simulink model "CSD_Segway_Nonlinear"  (R2018b)
settings: Solver=ode5  StartTime=0.0  StopTime=10  FixedStep=1e-4  RelTol=1e-3
values from neighbouring files (symbols this model uses):
  alpha = n * k_t / R_m    (= 0.0446559297218)    [CSD_project.m]
  beta = n * k_t * k_b /R_m + f_m    (= 0.0270286969253)    [CSD_project.m]
  f_w = 0    [CSD_project.m]
  g = 9.81    [CSD_project.m]
  J_m = 10^(-5)    (= 1e-05)    [CSD_project.m]
  K = place(A, B, 1e2*[-5,      -1, -0.8, -0.8,      -2e-2, -2e-2])    [CSD_project.m]
  L = 0.125    [CSD_project.m]
  M = 0.6    [CSD_project.m]
  m_1 = (2 * m + M) * R^2 + 2 * J_w + 2 * n^2 * J_m    (= 0.00056096)    [CSD_project.m]
  m_3 = M * L^2 + J_psi + 2 * n^2 * J_m    (= 0.01252)    [CSD_project.m]
  m_4 = m * W^2 /2 + J_phi + W^2 / 2 / R^2 * (J_w + n^2 * J_m)    (= 0.00149726)    [CSD_project.m]
  n = 1    [CSD_project.m]
  R = 0.028    [CSD_project.m]
  W = 0.126    [CSD_project.m]
settings Model: Creator=sh  LastModifiedBy=sh

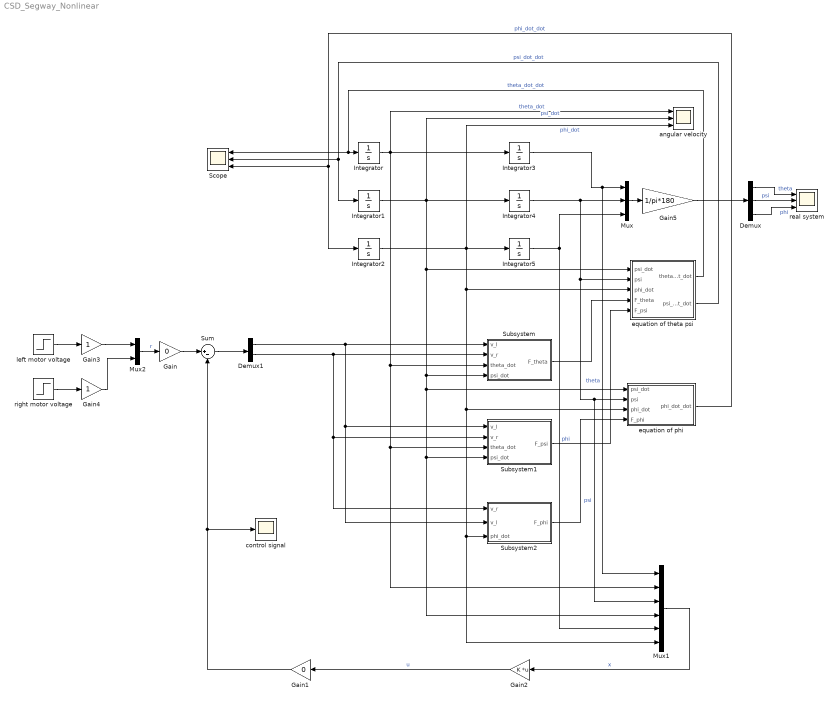
== system CSD_Segway_Nonlinear ==
  Demux : Demux  Outputs=3
  Demux1 : Demux  Outputs=2
  Gain : Gain  Gain=0
  Gain1 : Gain  Gain=0
  Gain2 : Gain  Gain=K  Multiplication=Matrix(K*u)
  Gain3 : Gain
  Gain4 : Gain
  Gain5 : Gain  Gain=1/pi*180
  Integrator : Integrator
  Integrator1 : Integrator
  Integrator2 : Integrator
  Integrator3 : Integrator  InitialCondition=pi
  Integrator4 : Integrator  InitialCondition=pi/36
  Integrator5 : Integrator  InitialCondition=pi/2
  Mux : Mux  Inputs=3
  Mux1 : Mux  Inputs=6
  Mux2 : Mux  Inputs=2
  Scope : Scope  NumInputPorts=3
  Subsystem : Subsystem
  Subsystem1 : Subsystem
  Subsystem2 : Subsystem
  Sum : Sum  Inputs=|+-
  angular velocity : Scope  NumInputPorts=3
  control signal : Scope
  equation of phi : Subsystem
  equation of theta psi : Subsystem
  left motor voltage : Step  SampleTime=0
  real system : Scope  NumInputPorts=3
  right motor voltage : Step  SampleTime=0
  wires:
  Integrator3/1 -> Mux1/1, Mux/1  "theta"
  Subsystem2/1(F_phi) -> equation of phi/4(F_phi)
  Subsystem/1(F_theta) -> equation of theta psi/4(F_theta)
  Integrator2/1 -> angular velocity/3, equation of theta psi/3(phi_dot), equation of phi/3(phi_dot), Mux1/6, Subsystem2/3(phi_dot), Integrator5/1  "phi_dot"
  Integrator/1 -> angular velocity/1, Mux1/2, Subsystem1/3(theta_dot), Subsystem/3(theta_dot), Integrator3/1  "theta_dot"
  equation of theta psi/2(psi_dot_dot) -> Integrator1/1, Scope/2  "psi_dot_dot"
  equation of theta psi/1(theta_dot_dot) -> Scope/1, Integrator/1  "theta_dot_dot"
  Integrator1/1 -> angular velocity/2, equation of theta psi/1(psi_dot), equation of phi/1(psi_dot), Mux1/4, Subsystem1/4(psi_dot), Subsystem/4(psi_dot), Integrator4/1  "psi_dot"
  Demux1/2 -> Subsystem2/1(v_r), Subsystem1/2(v_r), Subsystem/2(v_r)
  equation of phi/1(phi_dot_dot) -> Integrator2/1, Scope/3  "phi_dot_dot"
  Integrator4/1 -> Mux/2, Mux1/3, equation of phi/2(psi), equation of theta psi/2(psi)  "psi"
  Demux1/1 -> Subsystem1/1(v_l), Subsystem2/2(v_l), Subsystem/1(v_l)
  Subsystem1/1(F_psi) -> equation of theta psi/5(F_psi)
  Integrator5/1 -> Mux/3, Mux1/5  "phi"
  Mux1/1 -> Gain2/1  "x"
  Mux2/1 -> Gain/1  "r"
  left motor voltage/1 -> Gain3/1
  right motor voltage/1 -> Gain4/1
  Sum/1 -> Demux1/1
  Gain2/1 -> Gain1/1  "u"
  Gain/1 -> Sum/1
  Gain1/1 -> control signal/1, Sum/2
  Gain3/1 -> Mux2/1
  Gain4/1 -> Mux2/2
  Demux/1 -> real system/1  "theta"
  Demux/2 -> real system/2  "psi"
  Demux/3 -> real system/3  "phi"
  Mux/1 -> Gain5/1
  Gain5/1 -> Demux/1

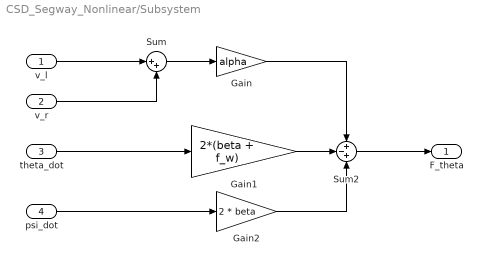
== system CSD_Segway_Nonlinear/Subsystem ==
  v_l : Inport
  v_r : Inport  Port=2
  theta_dot : Inport  Port=3
  psi_dot : Inport  Port=4
  Gain : Gain  Gain=alpha
  Gain1 : Gain  Gain=2*(beta + f_w)
  Gain2 : Gain  Gain=2 * beta
  Sum : Sum  Inputs=|++
  Sum2 : Sum  Inputs=+-+
  F_theta : Outport
  wires:
  v_l/1 -> Sum/1
  theta_dot/1 -> Gain1/1
  v_r/1 -> Sum/2
  Sum2/1 -> F_theta/1
  Gain1/1 -> Sum2/2
  Gain/1 -> Sum2/1
  Sum/1 -> Gain/1
  psi_dot/1 -> Gain2/1
  Gain2/1 -> Sum2/3

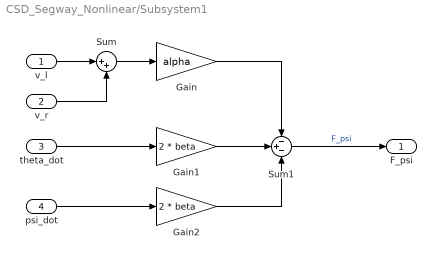
== system CSD_Segway_Nonlinear/Subsystem1 ==
  v_l : Inport
  v_r : Inport  Port=2
  theta_dot : Inport  Port=3
  psi_dot : Inport  Port=4
  Gain : Gain  Gain=alpha
  Gain1 : Gain  Gain=2 * beta
  Gain2 : Gain  Gain=2 * beta
  Sum : Sum  Inputs=|++
  Sum1 : Sum  Inputs=-+-
  F_psi : Outport
  wires:
  psi_dot/1 -> Gain2/1
  v_l/1 -> Sum/1
  Sum/1 -> Gain/1
  Sum1/1 -> F_psi/1  "F_psi"
  theta_dot/1 -> Gain1/1
  Gain/1 -> Sum1/1
  v_r/1 -> Sum/2
  Gain2/1 -> Sum1/3
  Gain1/1 -> Sum1/2

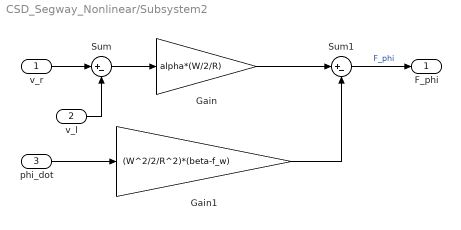
== system CSD_Segway_Nonlinear/Subsystem2 ==
  v_r : Inport
  v_l : Inport  Port=2
  phi_dot : Inport  Port=3
  Gain : Gain  Gain=alpha*(W/2/R)
  Gain1 : Gain  Gain=(W^2/2/R^2)*(beta-f_w)
  Sum : Sum  Inputs=|+-
  Sum1 : Sum  Inputs=|+-
  F_phi : Outport
  wires:
  Sum1/1 -> F_phi/1  "F_phi"
  phi_dot/1 -> Gain1/1
  v_l/1 -> Sum/2
  v_r/1 -> Sum/1
  Sum/1 -> Gain/1
  Gain/1 -> Sum1/1
  Gain1/1 -> Sum1/2

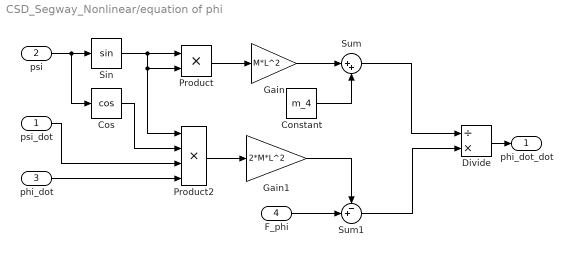
== system CSD_Segway_Nonlinear/equation of phi ==
  psi_dot : Inport
  psi : Inport  Port=2
  phi_dot : Inport  Port=3
  F_phi : Inport  Port=4
  Constant : Constant  Value=m_4
  Cos : Trigonometry  Operator=cos
  Divide : Product  Inputs=/*
  Gain : Gain  Gain=M*L^2
  Gain1 : Gain  Gain=2*M*L^2
  Product : Product
  Product2 : Product  Inputs=4
  Sin : Trigonometry
  Sum : Sum  Inputs=|++
  Sum1 : Sum  Inputs=-+|
  phi_dot_dot : Outport
  wires:
  psi_dot/1 -> Product2/3
  F_phi/1 -> Sum1/2
  Gain/1 -> Sum/1
  Constant/1 -> Sum/2
  Product2/1 -> Gain1/1
  Sum/1 -> Divide/1
  Gain1/1 -> Sum1/1
  psi/1 -> Cos/1, Sin/1
  Product/1 -> Gain/1
  Sum1/1 -> Divide/2
  phi_dot/1 -> Product2/4
  Cos/1 -> Product2/2
  Divide/1 -> phi_dot_dot/1
  Sin/1 -> Product/2, Product2/1, Product/1

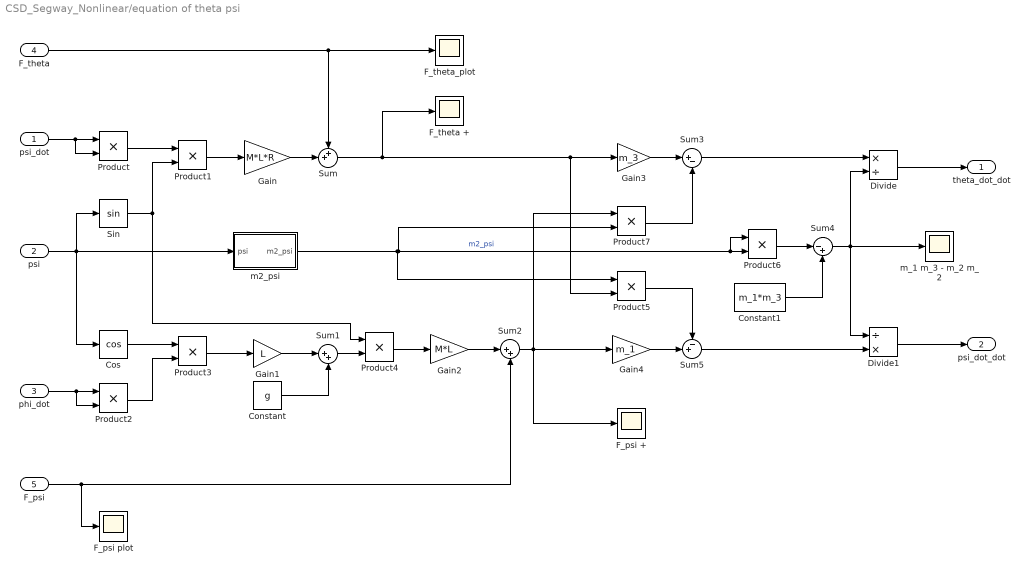
== system CSD_Segway_Nonlinear/equation of theta psi ==
  psi_dot : Inport
  psi : Inport  Port=2
  phi_dot : Inport  Port=3
  F_theta : Inport  Port=4
  F_psi : Inport  Port=5
  Constant : Constant  Value=g
  Constant1 : Constant  Value=m_1*m_3
  Cos : Trigonometry  Operator=cos
  Divide : Product  Inputs=*/
  Divide1 : Product  Inputs=/*
  "F_psi + " : Scope
  F_psi plot : Scope
  F_theta + : Scope
  F_theta_plot : Scope
  Gain : Gain  Gain=M*L*R
  Gain1 : Gain  Gain=L
  Gain2 : Gain  Gain=M*L
  Gain3 : Gain  Gain=m_3
  Gain4 : Gain  Gain=m_1
  Product{,1..7} (8 alike) : Product
  Sin : Trigonometry
  Sum : Sum  Inputs=++|
  Sum1 : Sum  Inputs=|++
  Sum2 : Sum  Inputs=|++
  Sum3 : Sum  Inputs=|+-
  Sum4 : Sum  Inputs=|-+
  Sum5 : Sum  Inputs=-+|
  m2_psi : Subsystem
  m_1 m_3 - m_2 m_2 : Scope
  theta_dot_dot : Outport
  psi_dot_dot : Outport  Port=2
  wires:
  Product2/1 -> Product3/2
  Product4/1 -> Gain2/1
  Gain2/1 -> Sum2/1
  Gain1/1 -> Sum1/1
  psi/1 -> Cos/1, m2_psi/1(psi), Sin/1
  F_psi/1 -> F_psi plot/1, Sum2/2
  Product3/1 -> Gain1/1
  Sum1/1 -> Product4/2
  phi_dot/1 -> Product2/2, Product2/1
  Product1/1 -> Gain/1
  psi_dot/1 -> Product/2, Product/1
  Cos/1 -> Product3/1
  Product/1 -> Product1/1
  Constant/1 -> Sum1/2
  Sum/1 -> F_theta +/1, Product5/2, Gain3/1
  Sum2/1 -> "F_psi + "/1, Product7/1, Gain4/1
  Gain3/1 -> Sum3/1
  Product7/1 -> Sum3/2
  Sum3/1 -> Divide/1
  Product6/1 -> Sum4/1
  Constant1/1 -> Sum4/2
  m2_psi/1(m2_psi) -> Product6/1, Product6/2, Product7/2, Product5/1  "m2_psi"
  Gain4/1 -> Sum5/2
  Product5/1 -> Sum5/1
  Sum5/1 -> Divide1/2
  Divide/1 -> theta_dot_dot/1
  Divide1/1 -> psi_dot_dot/1
  Gain/1 -> Sum/2
  F_theta/1 -> Sum/1, F_theta_plot/1
  Sin/1 -> Product1/2, Product4/1
  Sum4/1 -> m_1 m_3 - m_2 m_2/1, Divide1/1, Divide/2

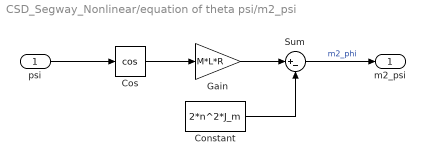
== system CSD_Segway_Nonlinear/equation of theta psi/m2_psi ==
  psi : Inport
  Constant : Constant  Value=2*n^2*J_m
  Cos : Trigonometry  Operator=cos
  Gain : Gain  Gain=M*L*R
  Sum : Sum  Inputs=|+-
  m2_psi : Outport
  wires:
  Gain/1 -> Sum/1
  psi/1 -> Cos/1
  Sum/1 -> m2_psi/1  "m2_phi"
  Cos/1 -> Gain/1
  Constant/1 -> Sum/2
